simulink library "sensor_processing_libs"  (R2016b)
settings: Solver=VariableStepAuto  StartTime=0.0  StopTime=10.0  RelTol=1e-3
undefined symbols (not defined in the file or in its folder): fsw_params
libraries: simulink x2, ss_angles_2_vec x1
settings Model: Creator=taylorreynolds  LastModifiedBy=Taylor

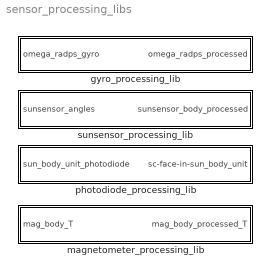
== system sensor_processing_libs ==
  gyro_processing_lib : Subsystem
  magnetometer_processing_lib : Subsystem
  photodiode_processing_lib : Subsystem
  sunsensor_processing_lib : Subsystem

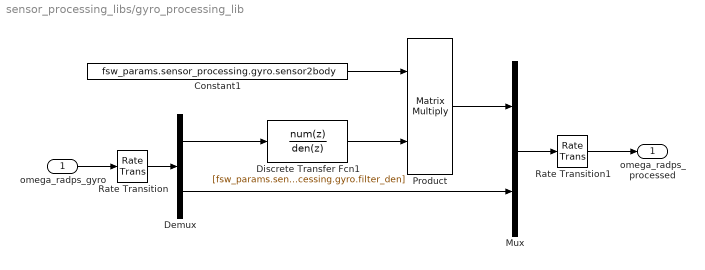
== system sensor_processing_libs/gyro_processing_lib ==
  omega_radps_gyro : Inport
  Constant1 : Constant  Value=fsw_params.sensor_processing.gyro.sensor2body  SampleTime=fsw_params.sensor_processing.gyro.sample_time_s
  Demux : Demux  Outputs=[3 1]
  Discrete Transfer Fcn1 : DiscreteTransferFcn  Numerator=[fsw_params.sensor_processing.gyro.filter_num]  Denominator=[1 fsw_params.sensor_processing.gyro.filter_den]
  Mux : Mux  Inputs=[3 1]
  Product : Product  Multiplication=Matrix(*)
  Rate Transition : RateTransition  OutPortSampleTime=fsw_params.sensor_processing.gyro.sample_time_s
  Rate Transition1 : RateTransition
  omega_radps_processed : Outport
  wires:
  omega_radps_gyro/1 -> Rate Transition/1
  Demux/1 -> Discrete Transfer Fcn1/1
  Constant1/1 -> Product/1
  Product/1 -> Mux/1
  Demux/2 -> Mux/2
  Mux/1 -> Rate Transition1/1
  Discrete Transfer Fcn1/1 -> Product/2
  Rate Transition/1 -> Demux/1
  Rate Transition1/1 -> omega_radps_processed/1

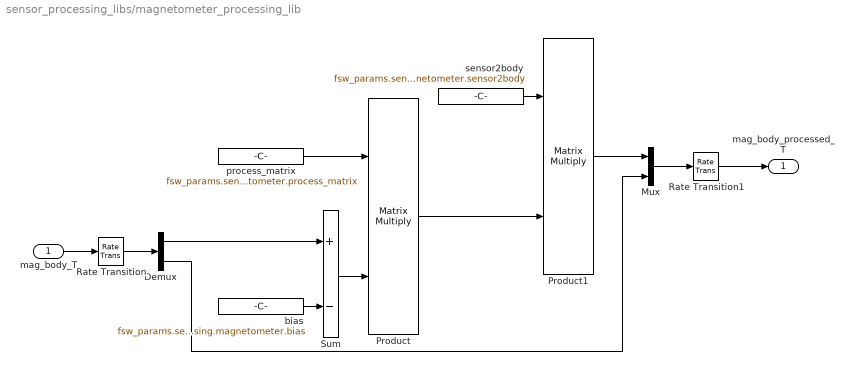
== system sensor_processing_libs/magnetometer_processing_lib ==
  mag_body_T : Inport
  Demux : Demux  Outputs=[3 1]
  Mux : Mux  Inputs=[3 1]
  Product : Product  Multiplication=Matrix(*)
  Product1 : Product  Multiplication=Matrix(*)
  Rate Transition : RateTransition  OutPortSampleTime=fsw_params.sensor_processing.magnetometer.sample_time_s
  Rate Transition1 : RateTransition
  Sum : Sum  Inputs=+-
  bias : Constant  Value=fsw_params.sensor_processing.magnetometer.bias  SampleTime=fsw_params.sensor_processing.magnetometer.sample_time_s
  process_matrix : Constant  Value=fsw_params.sensor_processing.magnetometer.process_matrix  SampleTime=fsw_params.sensor_processing.magnetometer.sample_time_s
  sensor2body : Constant  Value=fsw_params.sensor_processing.magnetometer.sensor2body  SampleTime=fsw_params.sensor_processing.magnetometer.sample_time_s
  mag_body_processed_T : Outport
  wires:
  mag_body_T/1 -> Rate Transition/1
  bias/1 -> Sum/2
  Sum/1 -> Product/2
  process_matrix/1 -> Product/1
  Demux/1 -> Sum/1
  Demux/2 -> Mux/2
  Mux/1 -> Rate Transition1/1
  Product/1 -> Product1/2
  sensor2body/1 -> Product1/1
  Product1/1 -> Mux/1
  Rate Transition/1 -> Demux/1
  Rate Transition1/1 -> mag_body_processed_T/1

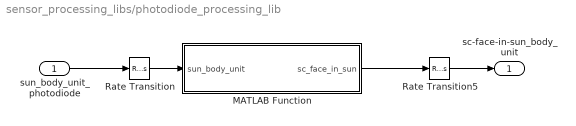
== system sensor_processing_libs/photodiode_processing_lib ==
  sun_body_unit_photodiode : Inport
  MATLAB Function : MATLAB Function  TreatAsAtomicUnit=on
  Rate Transition : RateTransition  OutPortSampleTime=fsw_params.sensor_processing.photodiodes.sample_time_s
  Rate Transition5 : RateTransition
  sc-face-in-sun_body_unit : Outport
  wires:
  sun_body_unit_photodiode/1 -> Rate Transition/1
  MATLAB Function/1(sc_face_in_sun) -> Rate Transition5/1
  Rate Transition/1 -> MATLAB Function/1(sun_body_unit)
  Rate Transition5/1 -> sc-face-in-sun_body_unit/1

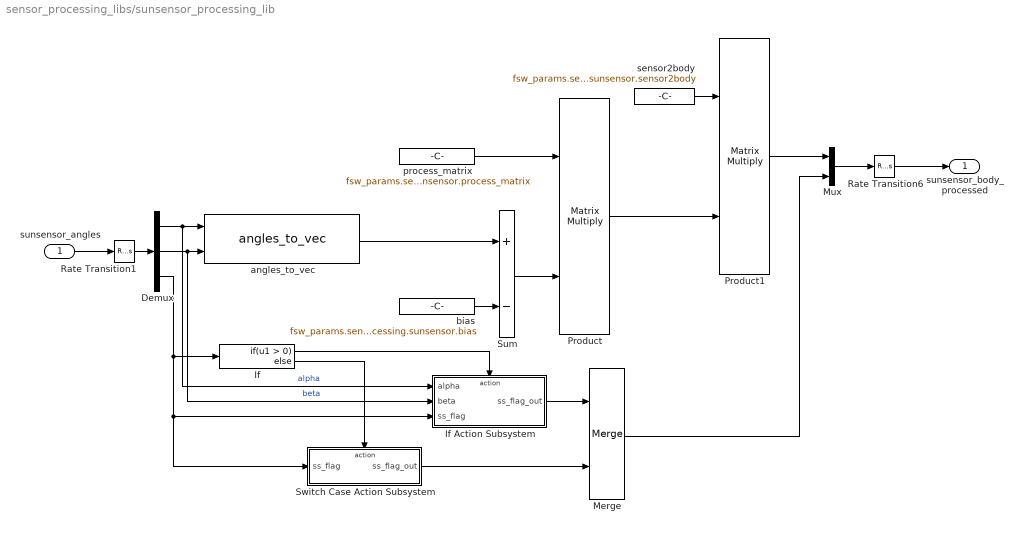
== system sensor_processing_libs/sunsensor_processing_lib ==
  sunsensor_angles : Inport
  Demux : Demux  Outputs=[1 1 1]
  If : If
  If Action Subsystem : Subsystem  TreatAsAtomicUnit=on
  Merge : Merge
  Mux : Mux  Inputs=[3 1]
  Product : Product  Multiplication=Matrix(*)
  Product1 : Product  Multiplication=Matrix(*)
  Rate Transition1 : RateTransition  X0=fsw_params.sensor_processing.sunsensor.ic.angles  OutPortSampleTime=fsw_params.sensor_processing.sunsensor.sample_time_s
  Rate Transition6 : RateTransition
  Sum : Sum  Inputs=+-
  Switch Case Action Subsystem : Subsystem  TreatAsAtomicUnit=on
  angles_to_vec : ss_angles_2_vec/angles_to_vec
  bias : Constant  Value=fsw_params.sensor_processing.sunsensor.bias  SampleTime=fsw_params.sensor_processing.sunsensor.sample_time_s
  process_matrix : Constant  Value=fsw_params.sensor_processing.sunsensor.process_matrix  SampleTime=fsw_params.sensor_processing.sunsensor.sample_time_s
  sensor2body : Constant  Value=fsw_params.sensor_processing.sunsensor.sensor2body  SampleTime=fsw_params.sensor_processing.sunsensor.sample_time_s
  sunsensor_body_processed : Outport
  wires:
  Switch Case Action Subsystem/1(ss_flag_out) -> Merge/2
  If Action Subsystem/1(ss_flag_out) -> Merge/1
  If/2 -> Switch Case Action Subsystem/Action
  If/1 -> If Action Subsystem/Action
  Demux/3 -> If/1, Switch Case Action Subsystem/1(ss_flag), If Action Subsystem/3(ss_flag)
  Merge/1 -> Mux/2
  angles_to_vec/1 -> Sum/1
  Demux/2 -> angles_to_vec/2, If Action Subsystem/2(beta)  "beta"
  Demux/1 -> angles_to_vec/1, If Action Subsystem/1(alpha)  "alpha"
  Rate Transition6/1 -> sunsensor_body_processed/1
  Rate Transition1/1 -> Demux/1
  Mux/1 -> Rate Transition6/1
  Product1/1 -> Mux/1
  sensor2body/1 -> Product1/1
  sunsensor_angles/1 -> Rate Transition1/1
  bias/1 -> Sum/2
  Product/1 -> Product1/2
  Sum/1 -> Product/2
  process_matrix/1 -> Product/1

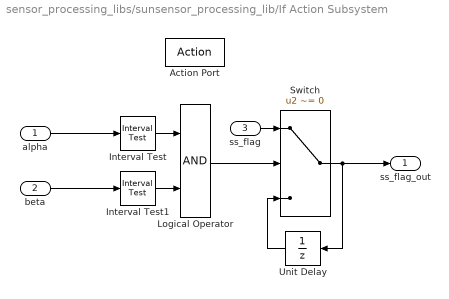
== system sensor_processing_libs/sunsensor_processing_lib/If Action Subsystem ==
  alpha : Inport
  beta : Inport  Port=2
  ss_flag : Inport  Port=3
  Action Port : ActionPort  InitializeStates=reset
  Interval Test : simulink/Logic and Bit Operations/Interval Test  IntervalClosedRight=on  uplimit=fsw_params.sensor_processing.sunsensor.ang_thresh  IntervalClosedLeft=on  lowlimit=-fsw_params.sensor_processing.sunsensor.ang_thresh  OutDataTypeStr=boolean
  Interval Test1 : simulink/Logic and Bit Operations/Interval Test  IntervalClosedRight=on  uplimit=fsw_params.sensor_processing.sunsensor.ang_thresh  IntervalClosedLeft=on  lowlimit=-fsw_params.sensor_processing.sunsensor.ang_thresh  OutDataTypeStr=boolean
  Logical Operator : Logic  AllPortsSameDT=off  OutDataTypeStr=boolean
  Switch : Switch  Criteria=u2 ~= 0
  Unit Delay : UnitDelay  InitialCondition=2  SampleTime=fsw_params.sensor_processing.sunsensor.sample_time_s
  ss_flag_out : Outport
  wires:
  Unit Delay/1 -> Switch/3
  Logical Operator/1 -> Switch/2
  ss_flag/1 -> Switch/1
  alpha/1 -> Interval Test/1
  beta/1 -> Interval Test1/1
  Interval Test1/1 -> Logical Operator/2
  Interval Test/1 -> Logical Operator/1
  Switch/1 -> Unit Delay/1, ss_flag_out/1

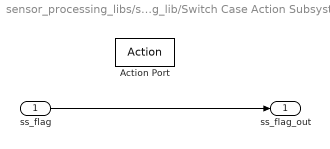
== system sensor_processing_libs/sunsensor_processing_lib/Switch Case Action Subsystem ==
  ss_flag : Inport
  Action Port : ActionPort
  ss_flag_out : Outport
  wires:
  ss_flag/1 -> ss_flag_out/1

== matlab function sensor_processing_libs/photodiode_processing_lib/MATLAB Function ==
  data: sun_body_unit input; sc_face_in_sun output
 function sc_face_in_sun = fcn(sun_body_unit)

body_vecs   = [ 1  0  0;
                0  1  0;
                0  0  1;
               -1  0  0;
                0 -1  0 ];
            
num_faces = 5;
dot_prods   = zeros(1,5);

for i = 1:num_faces
    dot_prods(i)    = dot(sun_body_unit,body_vecs(i,:));
end

[val,axis] = max(dot_prods);

if val < 0
    % this is only the case if the PPT is pointing right at the sun
    sc_face_in_sun = [ 0 0 -1 ]';
else
    sc_face_in_sun  = body_vecs(axis,:)';
end
